simulink model "Standalone_EncoderGeneration"  (R2023b)
settings: Solver=FixedStepAuto  StartTime=0.0  StopTime=inf  RelTol=1e-3
undefined symbols (not defined in the file): DiscIntNeverNeededParam, IO397
libraries: simulink x2, speedgoatlib_fpga_dio x1, speedgoatlib_fpga x1
settings Model: PacingRate=0.010000  Creator=rodri  LastModifiedBy=rodri
settings SolverCC: ConcurrentTasks=on  PositivePriorityOrder=on
settings OptimizationCC: BlockReduction=off  OptimizeBlockIOStorage=off
settings DebuggingCC: TasksWithSamePriorityMsg=none
settings HardwareCC: ProdBitPerLong=64  ProdLongLongMode=on  ProdHWDeviceType=Intel->x86-64 (Linux 64)
settings RTWCC: Description=Simulink Real-Time  SystemTargetFile=slrealtime.tlc  TemplateMakefile=slrealtime_default_tmf  Toolchain=Simulink Real-Time Toolchain  BuildConfiguration=Faster Runs  CodeExecutionProfiling=on  TargetLang=C++

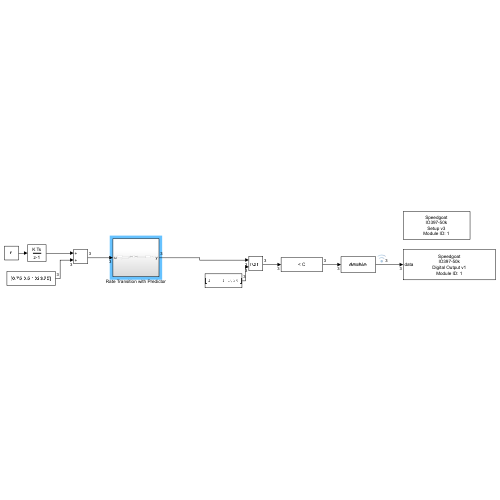
[thumbnail: Simulink's stored preview of the top-level diagram]
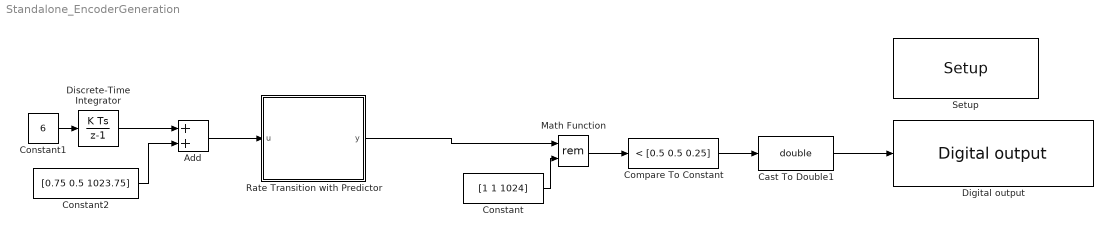
== system Standalone_EncoderGeneration ==
  Add : Sum
  Cast To Double1 : DataTypeConversion  OutDataTypeStr=double  SaturateOnIntegerOverflow=off  RndMeth=Floor
  Compare To Constant : simulink/Logic and Bit Operations/Compare To Constant  relop=<  const=[0.5 0.5 0.25]  OutDataTypeStr=boolean
  Constant : Constant  Value=[1 1 1024]
  Constant1 : Constant  Value=6  SampleTime=0.001
  Constant2 : Constant  Value=[0.75 0.5 1023.75]  SampleTime=-1
  Digital output : speedgoatlib_fpga_dio/Digital output  id=1  chan=[9:11]  init=[0]  reset=[0]  ts=0.0001  vectorizeInput=on
      settings: SourceProductName=Simulink Real-Time: Speedgoat I/O Blockset
  Discrete-Time Integrator : DiscreteIntegrator  gainval=1024/(2*pi)  SampleTime=-1  ICPrevOutput=DiscIntNeverNeededParam  ICPrevScaledInput=DiscIntNeverNeededParam
  Math Function : Math  Operator=rem  SignedPower=on  RndMeth=Zero
  Rate Transition with Predictor : Subsystem
  Setup : speedgoatlib_fpga/Setup/Setup  board=IO397-50k  id=1  device_id=1  frontIO=None  rearIO=None  bitstreamFile=speedgoat_IO397_HIL.mat  rev=7.100000  timestamp_string=04/06/24 08:23:17  fpgaFreq=75 MHz  fpgaTick=13.33 ns  ProgSpiFlash=off  ProgBPIFlash=off  pciSlot=-1  useFpgaDmaController=off  PullRPort0=pull-up 3.3V  VioPort0=3.3V  PullRPort1=pull-up 3.3V  VioPort1=3.3V  PullRPort2=pull-up 3.3V  VioPort2=3.3V  PullRPort3=pull-up 3.3V  VioPort3=3.3V  PullRPort4=pull-up 3.3V  VioPort4=3.3V  PullRPort5=pull-up 3.3V  VioPort5=3.3V  PullRPort6=pull-up 3.3V  VioPort6=3.3V  diffLineTermination_rear1=on  diffLineTermination_rear2=on  diffLineTermination_rear3=on  diffLineTermination_rear4=on  diffLineTermination_rear5=on  diffLineTermination_rear6=on  diffLineTermination_rear7=on  diffLineTermination_rear8=on  PullRPort15=pull-up 3.3V  PullRPort31=pull-up 3.3V  PullRPort47=pull-up 3.3V  PullRPort63=pull-up 3.3V  diffLineTermination_1=on  diffLineTermination_2=on  diffLineTermination_3=on  diffLineTermination_4=on  diffLineTermination_5=on  diffLineTermination_6=on  diffLineTermination_7=on  diffLineTermination_8=on  diffLineTermination_9=on  diffLineTermination_10=on  diffLineTermination_11=on  diffLineTermination_12=on  diffLineTermination_13=on  diffLineTermination_14=on  diffLineTermination_15=on  diffLineTermination_16=on  diffLineTermination_17=on  diffLineTermination_18=on  diffLineTermination_19=on  diffLineTermination_20=on  diffLineTermination_21=on  diffLineTermination_22=on  diffLineTermination_23=on  diffLineTermination_24=on  diffLineTermination_25=on  diffLineTermination_26=on  diffLineTermination_27=on  diffLineTermination_28=on  diffLineTermination_29=on  diffLineTermination_30=on  diffLineTermination_31=on  diffLineTermination_32=on  Vo_36x_1=3.3V  Vi_Pull_36x_1=Floating  Vo_36x_2=3.3V  Vi_Pull_36x_2=Floating  Vo_36x_3=3.3V  Vi_Pull_36x_3=Floating  Vo_36x_4=3.3V  Vi_Pull_36x_4=Floating  Vo_36x_5=3.3V  Vi_Pull_36x_5=Floating  Vo_36x_6=3.3V  Vi_Pull_36x_6=Floating  Vo_36x_7=3.3V  Vi_Pull_36x_7=Floating  Vo_36x_8=3.3V  Vi_Pull_36x_8=Floating  Vo_36x_9_16=3.3V  Vi_Pull_36x_9_16=Floating  Vo_36x_17_24=3.3V  Vi_Pull_36x_17_24=Floating  Vo_36x_25_32=3.3V  Vi_Pull_36x_25_32=Floating  Vo_36x_33_40=3.3V  Vi_Pull_36x_33_40=Floating  Vo_36x_41_48=3.3V  Vi_Pull_36x_41_48=Floating  Vo_36x_49_56=3.3V  Vi_Pull_36x_49_56=Floating  Vo_36x_57_64=3.3V  Vi_Pull_36x_57_64=Floating
      settings: SourceProductName=Simulink Real-Time: Speedgoat I/O Blockset
  wires:
  Discrete-Time Integrator/1 -> Add/1
  Constant/1 -> Math Function/2
  Math Function/1 -> Compare To Constant/1
  Constant1/1 -> Discrete-Time Integrator/1
  Compare To Constant/1 -> Cast To Double1/1
  Cast To Double1/1 -> Digital output/1
  Constant2/1 -> Add/2
  Add/1 -> Rate Transition with Predictor/1(u)
  Rate Transition with Predictor/1(y) -> Math Function/1

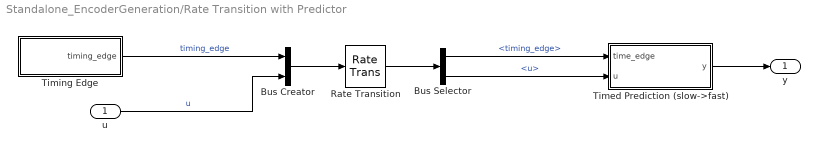
== system Standalone_EncoderGeneration/Rate Transition with Predictor ==
  u : Inport
  Bus Creator : BusCreator  Inputs=2
  Bus Selector : BusSelector  OutputSignals=timing_edge,u
  Rate Transition : RateTransition
  Timed Prediction (slow->fast) : Subsystem  mask(Prediction (slow->fast)){h2=0.001, h1=0.0001}
      mask prompts: h2 "physmod:simscape:couplers:SimscapeNetworkCouplersLib:PortUDiscreteSampleTimes_MP"; h1 "physmod:simscape:couplers:SimscapeNetworkCouplersLib:PortYDiscreteSampleTimes_MP"
      mask help: physmod:simscape:couplers:SimscapeNetworkCouplersLib:Predictionslowfast_MD
      mask Help: web([docroot '/simscape/ref/predictionslowfast.html'])
      mask DialogControl h2 Prompt: Port u discrete sample time (s)
      mask DialogControl h1 Prompt: Port y discrete sample time (s)
  Timing Edge : Subsystem
  y : Outport
  wires:
  Timed Prediction (slow->fast)/1(y) -> y/1
  Bus Creator/1 -> Rate Transition/1
  Rate Transition/1 -> Bus Selector/1
  Bus Selector/1 -> Timed Prediction (slow->fast)/1(time_edge)  "<timing_edge>"
  Bus Selector/2 -> Timed Prediction (slow->fast)/2(u)  "<u>"
  Timing Edge/1(timing_edge) -> Bus Creator/1  "timing_edge"
  u/1 -> Bus Creator/2  "u"

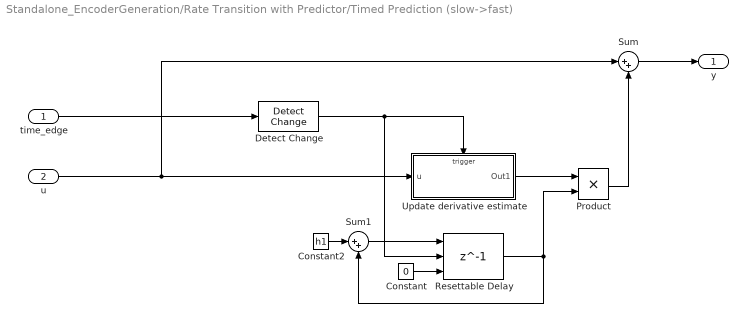
== system Standalone_EncoderGeneration/Rate Transition with Predictor/Timed Prediction (slow->fast) ==
  time_edge : Inport
  u : Inport  Port=2
  Constant : Constant  Value=0  SampleTime=h1
  Constant2 : Constant  Value=h1  SampleTime=h1
  Detect Change : simulink/Logic and Bit Operations/Detect Change  vinit=0  OutDataTypeStr=boolean
  Product : Product
  Resettable Delay : Delay  DelayLength=1  InitialConditionSource=Input port  ExternalReset=Rising  SampleTime=h1
      settings: InputPortMap=u0,r5,p4
  Sum : Sum  Inputs=|++
  Sum1 : Sum  Inputs=|++
  Update derivative estimate : Subsystem  TreatAsAtomicUnit=on
  y : Outport
  wires:
  Product/1 -> Sum/2
  Sum/1 -> y/1
  Constant/1 -> Resettable Delay/3
  Constant2/1 -> Sum1/1
  Resettable Delay/1 -> Sum1/2, Product/2
  Sum1/1 -> Resettable Delay/1
  Update derivative estimate/1(Out1) -> Product/1
  Detect Change/1 -> Resettable Delay/2, Update derivative estimate/Trigger
  u/1 -> Sum/1, Update derivative estimate/1(u)
  time_edge/1 -> Detect Change/1

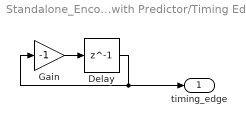
== system Standalone_EncoderGeneration/Rate Transition with Predictor/Timing Edge ==
  Delay : Delay  DelayLength=1  InitialCondition=1  UseCircularBuffer=on  SampleTime=0.001
  Gain : Gain  Gain=-1
  timing_edge : Outport
  wires:
  Gain/1 -> Delay/1
  Delay/1 -> timing_edge/1, Gain/1

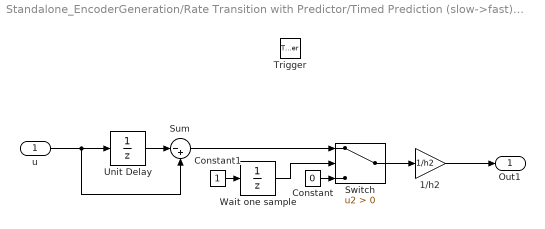
== system Standalone_EncoderGeneration/Rate Transition with Predictor/Timed Prediction (slow->fast)/Update derivative estimate ==
  u : Inport
  Trigger : TriggerPort  VariantControl=(inherit)
  1/h2 : Gain  Gain=1/h2
  Constant : Constant  Value=0  SampleTime=-1
  Constant1 : Constant  SampleTime=-1
  Sum : Sum  Inputs=|-+
  Switch : Switch  Criteria=u2 > Threshold  SaturateOnIntegerOverflow=off  InputSameDT=off
  Unit Delay : UnitDelay  SampleTime=-1  HasFrameUpgradeWarning=on
  Wait one sample : UnitDelay  SampleTime=-1  HasFrameUpgradeWarning=on
  Out1 : Outport
  wires:
  Unit Delay/1 -> Sum/1
  u/1 -> Unit Delay/1, Sum/2
  1/h2/1 -> Out1/1
  Switch/1 -> 1/h2/1
  Sum/1 -> Switch/1
  Constant/1 -> Switch/3
  Wait one sample/1 -> Switch/2
  Constant1/1 -> Wait one sample/1
